simulink library "sunsensor_processing_lib"  (R2018b)
settings: Solver=VariableStepAuto  StartTime=0.0  StopTime=10.0  RelTol=1e-3
undefined symbols (not defined in the file or in its folder): fswParams, simParams
libraries: simulink x2
settings Model: Creator=Taylor  LastModifiedBy=Taylor

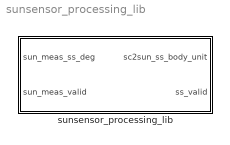
== system sunsensor_processing_lib ==
  sunsensor_processing_lib : Subsystem

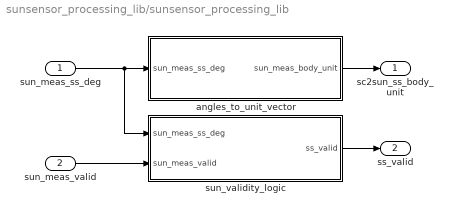
== system sunsensor_processing_lib/sunsensor_processing_lib ==
  sun_meas_ss_deg : Inport
  sun_meas_valid : Inport  Port=2
  angles_to_unit_vector : Subsystem
  sun_validity_logic : Subsystem
  sc2sun_ss_body_unit : Outport
  ss_valid : Outport  Port=2
  wires:
  sun_meas_ss_deg/1 -> sun_validity_logic/1(sun_meas_ss_deg), angles_to_unit_vector/1(sun_meas_ss_deg)
  sun_meas_valid/1 -> sun_validity_logic/2(sun_meas_valid)
  sun_validity_logic/1(ss_valid) -> ss_valid/1
  angles_to_unit_vector/1(sun_meas_body_unit) -> sc2sun_ss_body_unit/1

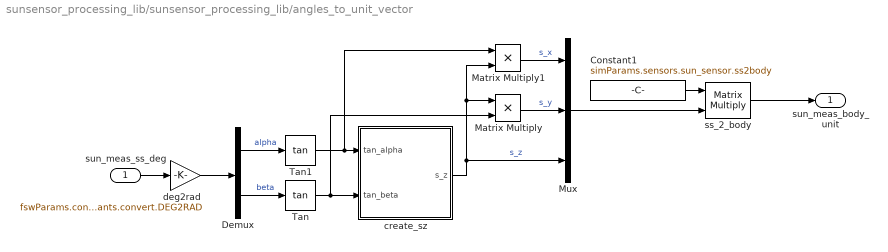
== system sunsensor_processing_lib/sunsensor_processing_lib/angles_to_unit_vector ==
  sun_meas_ss_deg : Inport
  Constant1 : Constant  Value=simParams.sensors.sun_sensor.ss2body
  Demux : Demux  Outputs=2
  Matrix Multiply : Product
  Matrix Multiply1 : Product
  Mux : Mux  Inputs=3
  Tan : Trigonometry  Operator=tan
  Tan1 : Trigonometry  Operator=tan
  create_sz : Subsystem
  deg2rad : Gain  Gain=fswParams.constants.convert.DEG2RAD
  ss_2_body : Product  Multiplication=Matrix(*)
  sun_meas_body_unit : Outport
  wires:
  sun_meas_ss_deg/1 -> deg2rad/1
  Demux/1 -> Tan1/1  "alpha"
  Matrix Multiply1/1 -> Mux/1  "s_x"
  Constant1/1 -> ss_2_body/1
  deg2rad/1 -> Demux/1
  Mux/1 -> ss_2_body/2
  Demux/2 -> Tan/1  "beta"
  Matrix Multiply/1 -> Mux/2  "s_y"
  ss_2_body/1 -> sun_meas_body_unit/1
  Tan1/1 -> create_sz/1(tan_alpha), Matrix Multiply1/1
  create_sz/1(s_z) -> Matrix Multiply/1, Matrix Multiply1/2, Mux/3  "s_z"
  Tan/1 -> Matrix Multiply/2, create_sz/2(tan_beta)

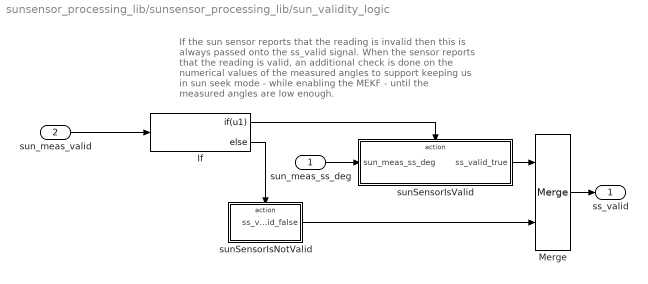
== system sunsensor_processing_lib/sunsensor_processing_lib/sun_validity_logic ==
  note: If the sun sensor reports that the reading is invalid
      | then this is always passed onto the ss_valid signal.
      | When the sensor reports that the reading is valid,
      | an additional check is done on the numerical values of
      | the measured angles to support keeping us in sun seek
      | mode - while enabling the MEKF - until the measured
      | angles are low enough.
  sun_meas_ss_deg : Inport
  sun_meas_valid : Inport  Port=2
  If : If  IfExpression=u1
  Merge : Merge
  sunSensorIsNotValid : Subsystem  TreatAsAtomicUnit=on
  sunSensorIsValid : Subsystem  TreatAsAtomicUnit=on
  ss_valid : Outport
  wires:
  sun_meas_valid/1 -> If/1
  If/1 -> sunSensorIsValid/Action
  If/2 -> sunSensorIsNotValid/Action
  sun_meas_ss_deg/1 -> sunSensorIsValid/1(sun_meas_ss_deg)
  sunSensorIsValid/1(ss_valid_true) -> Merge/1
  sunSensorIsNotValid/1(ss_valid_false) -> Merge/2
  Merge/1 -> ss_valid/1

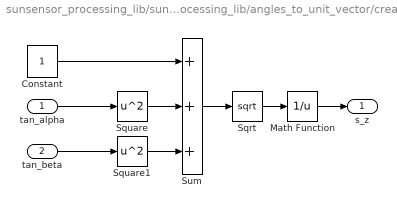
== system sunsensor_processing_lib/sunsensor_processing_lib/angles_to_unit_vector/create_sz ==
  tan_alpha : Inport
  tan_beta : Inport  Port=2
  Constant : Constant
  Math Function : Math  Operator=reciprocal  SaturateOnIntegerOverflow=on
  Sqrt : Sqrt  SaturateOnIntegerOverflow=on
  Square : Math  Operator=square  SaturateOnIntegerOverflow=on
  Square1 : Math  Operator=square  SaturateOnIntegerOverflow=on
  Sum : Sum  Inputs=+++
  s_z : Outport
  wires:
  tan_alpha/1 -> Square/1
  tan_beta/1 -> Square1/1
  Constant/1 -> Sum/1
  Square/1 -> Sum/2
  Square1/1 -> Sum/3
  Sum/1 -> Sqrt/1
  Sqrt/1 -> Math Function/1
  Math Function/1 -> s_z/1

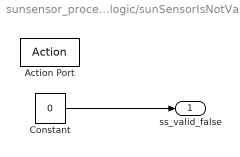
== system sunsensor_processing_lib/sunsensor_processing_lib/sun_validity_logic/sunSensorIsNotValid ==
  Action Port : ActionPort  ActionType=else
  Constant : Constant  Value=0  OutDataTypeStr=uint8
  ss_valid_false : Outport
  wires:
  Constant/1 -> ss_valid_false/1

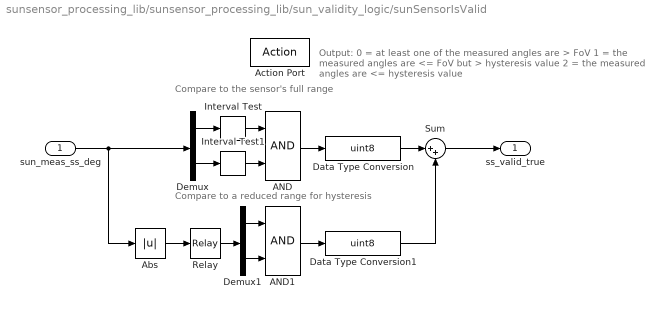
== system sunsensor_processing_lib/sunsensor_processing_lib/sun_validity_logic/sunSensorIsValid ==
  note: Output:
      | 0 = at least one of the measured angles are > FoV
      | 1 = the measured angles are <= FoV but > hysteresis value
      | 2 = the measured angles are <= hysteresis value
  note: Compare to a reduced range for hysteresis
  note: Compare to the sensor's full range
  sun_meas_ss_deg : Inport
  Action Port : ActionPort  ActionType=then
  AND : Logic  OutDataTypeStr=boolean
  AND1 : Logic  OutDataTypeStr=boolean
  Abs : Abs
  Data Type Conversion : DataTypeConversion  OutDataTypeStr=uint8  RndMeth=Nearest
  Data Type Conversion1 : DataTypeConversion  OutDataTypeStr=uint8  RndMeth=Nearest
  Demux : Demux  Outputs=[1 1]
  Demux1 : Demux  Outputs=2
  Interval Test : simulink/Logic and Bit Operations/Interval Test  IntervalClosedRight=on  uplimit=fswParams.sensors.sun_sensor_range_deg  IntervalClosedLeft=on  lowlimit=-fswParams.sensors.sun_sensor_range_deg  OutDataTypeStr=boolean
  Interval Test1 : simulink/Logic and Bit Operations/Interval Test  IntervalClosedRight=on  uplimit=fswParams.sensors.sun_sensor_range_deg  IntervalClosedLeft=on  lowlimit=-fswParams.sensors.sun_sensor_range_deg  OutDataTypeStr=boolean
  Relay : Relay  OnSwitchValue=fswParams.sensors.sun_sensor_range_deg  OffSwitchValue=fswParams.sensors.sunseek_hysteresis_deg  OnOutputValue=false  OffOutputValue=true  OutDataTypeStr=boolean
  Sum : Sum  Inputs=|++
  ss_valid_true : Outport
  wires:
  Data Type Conversion/1 -> Sum/1
  Demux/2 -> Interval Test1/1
  sun_meas_ss_deg/1 -> Demux/1, Abs/1
  AND/1 -> Data Type Conversion/1
  Demux/1 -> Interval Test/1
  Interval Test1/1 -> AND/2
  Data Type Conversion1/1 -> Sum/2
  AND1/1 -> Data Type Conversion1/1
  Interval Test/1 -> AND/1
  Sum/1 -> ss_valid_true/1
  Demux1/1 -> AND1/1
  Demux1/2 -> AND1/2
  Relay/1 -> Demux1/1
  Abs/1 -> Relay/1
